simulink model "MotorSysFin"  (R2019a)
settings: Solver=VariableStepAuto  StartTime=0.0  StopTime=10  RelTol=1e-3
libraries: fuzblock x2, simulink x1
settings Model: Creator=936305695  LastModifiedBy=936305695
settings SolverCC: AlgebraicLoopSolver=LineSearch

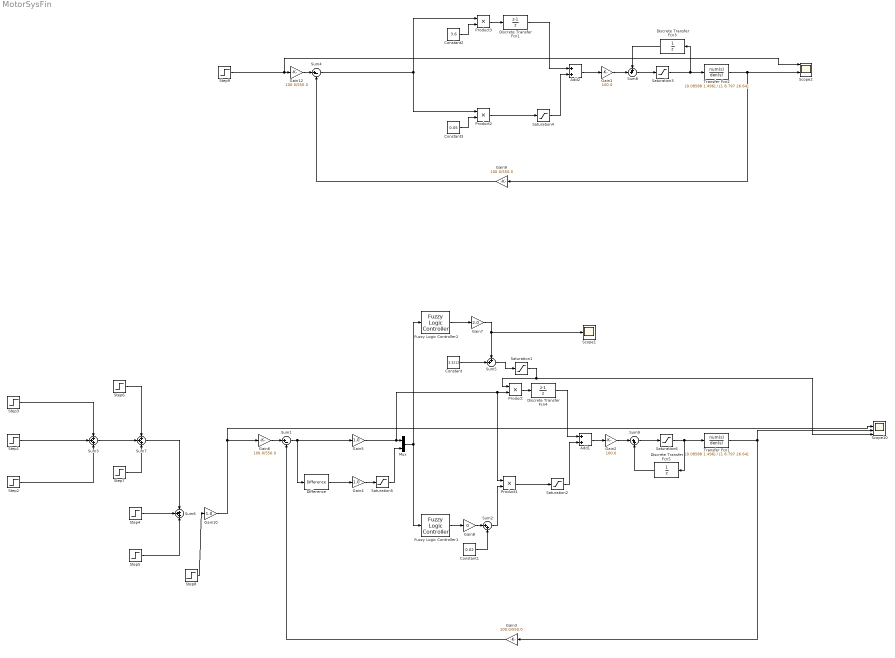
== system MotorSysFin ==
  Add1 : Sum
  Add2 : Sum
  Constant : Constant  Value=3.3212
  Constant1 : Constant  Value=0.02  SampleTime=0.002
  Constant2 : Constant  Value=3.6
  Constant3 : Constant  Value=0.05
  Difference : simulink/Discrete/Difference  ICPrevInput=0.0  OutMin=[]  OutMax=[]  OutDataType=fixdt(1, 16)  OutScaling=2^-10  DoSatur=off
  Discrete Transfer Fcn1 : DiscreteTransferFcn  Numerator=[1 -1]  Denominator=[1 0]  SampleTime=0.002
  Discrete Transfer Fcn3 : DiscreteTransferFcn  Denominator=[1 0]  SampleTime=0.002
  Discrete Transfer Fcn4 : DiscreteTransferFcn  Numerator=[1 -1]  Denominator=[1 0]  SampleTime=0.002
  Discrete Transfer Fcn5 : DiscreteTransferFcn  Denominator=[1 0]  SampleTime=0.002
  Fuzzy Logic Controller1 : fuzblock/Fuzzy Logic  Controller  FIS=mFuzzyKi  OutputSampleNumber=101  DataType=double  FuzzifiedInputs=off  RuleFiringStrengths=off  RuleOutputs=off  AggregatedOutputs=off  SimulateUsing=Interpreted execution  OutOfRangeInputValueMessage=warning  NoRuleFiredMessage=warning  EmptyOutputFuzzySetMessage=warning
  Fuzzy Logic Controller2 : fuzblock/Fuzzy Logic  Controller  FIS=mFuzzyKp  OutputSampleNumber=101  DataType=double  FuzzifiedInputs=off  RuleFiringStrengths=off  RuleOutputs=off  AggregatedOutputs=off  SimulateUsing=Interpreted execution  OutOfRangeInputValueMessage=warning  NoRuleFiredMessage=warning  EmptyOutputFuzzySetMessage=warning
  Gain1 : Gain  Gain=100.0
  Gain10 : Gain  Gain=1.0
  Gain{3,6,9,12} (4 alike) : Gain  Gain=100.0/550.0
  Gain2 : Gain  Gain=100.0
  Gain4 : Gain  Gain=1.0
  Gain5 : Gain  Gain=1.0
  Gain7 : Gain  Gain=2.0
  Gain8 : Gain  Gain=0
  Mux : Mux  Inputs=2
  Product{,1..3} (4 alike) : Product
  Saturation1 : Saturate  UpperLimit=20.0  LowerLimit=1.0
  Saturation2 : Saturate  UpperLimit=1.2  LowerLimit=-1.2
  Saturation3 : Saturate  UpperLimit=10000.0  LowerLimit=-10000.0
  Saturation4 : Saturate  UpperLimit=100  LowerLimit=-100
  Saturation5 : Saturate  UpperLimit=20.0  LowerLimit=-20.0
  Saturation6 : Saturate  UpperLimit=10000.0  LowerLimit=-10000.0
  Scope1 : Scope
  Scope10 : Scope  NumInputPorts=4
  Scope2 : Scope  NumInputPorts=4
  Step1 : Step  After=150  SampleTime=0
  Step2 : Step  Time=2  After=-100  SampleTime=0
  Step3 : Step  Time=3  After=100  SampleTime=0
  Step4 : Step  Time=6  After=-100  SampleTime=0
  Step5 : Step  Time=7  After=-50  SampleTime=0
  Step6 : Step  Time=4  After=-50  SampleTime=0
  Step7 : Step  Time=5  After=100  SampleTime=0
  Step8 : Step  After=150  SampleTime=0.002
  Step9 : Step  After=150  SampleTime=0.002
  Sum1 : Sum  Inputs=|+-
  Sum2 : Sum  Inputs=|++
  Sum3 : Sum  Inputs=+++
  Sum4 : Sum  Inputs=|+-
  Sum5 : Sum  Inputs=++|
  Sum6 : Sum  Inputs=+++
  Sum7 : Sum  Inputs=+++
  Sum8 : Sum  Inputs=++|
  Sum9 : Sum  Inputs=|++
  Transfer Fcn1 : TransferFcn  Numerator=[0.08588 1.496]  Denominator=[1 8.797 26.64]
  Transfer Fcn2 : TransferFcn  Numerator=[0.08588 1.496]  Denominator=[1 8.797 26.64]
  wires:
  Saturation2/1 -> Add1/2
  Product1/1 -> Saturation2/1
  Discrete Transfer Fcn4/1 -> Add1/1
  Transfer Fcn1/1 -> Scope10/3, Gain3/1
  Gain3/1 -> Sum1/2
  Sum1/1 -> Gain5/1, Difference/1
  Gain6/1 -> Sum1/1
  Mux/1 -> Fuzzy Logic Controller2/1, Fuzzy Logic Controller1/1
  Fuzzy Logic Controller2/1 -> Gain7/1
  Gain7/1 -> Sum5/1, Scope1/1
  Fuzzy Logic Controller1/1 -> Gain8/1
  Discrete Transfer Fcn1/1 -> Add2/1
  Product2/1 -> Saturation4/1
  Transfer Fcn2/1 -> Scope2/3, Gain9/1
  Gain9/1 -> Sum4/2
  Saturation4/1 -> Add2/2
  Gain12/1 -> Sum4/1
  Difference/1 -> Gain4/1
  Constant/1 -> Sum5/2
  Product/1 -> Discrete Transfer Fcn4/1
  Constant1/1 -> Sum2/2
  Gain8/1 -> Sum2/1
  Sum2/1 -> Product1/2
  Sum4/1 -> Product3/1, Product2/1
  Product3/1 -> Discrete Transfer Fcn1/1
  Gain4/1 -> Saturation5/1
  Gain10/1 -> Scope10/2, Gain6/1
  Saturation5/1 -> Mux/2
  Gain5/1 -> Product1/1, Product/2, Mux/1
  Step2/1 -> Sum3/3
  Step1/1 -> Sum3/2
  Step3/1 -> Sum3/1
  Step5/1 -> Sum6/3
  Step4/1 -> Sum6/2
  Sum3/1 -> Sum7/2
  Sum7/1 -> Sum6/1
  Step6/1 -> Sum7/1
  Step7/1 -> Sum7/3
  Sum5/1 -> Saturation1/1
  Saturation1/1 -> Scope10/4, Product/1
  Saturation3/1 -> Discrete Transfer Fcn3/1, Transfer Fcn2/1
  Add2/1 -> Gain1/1
  Gain1/1 -> Sum8/2
  Discrete Transfer Fcn3/1 -> Sum8/1
  Sum8/1 -> Saturation3/1
  Add1/1 -> Gain2/1
  Saturation6/1 -> Discrete Transfer Fcn5/1, Transfer Fcn1/1
  Sum9/1 -> Saturation6/1
  Gain2/1 -> Sum9/1
  Discrete Transfer Fcn5/1 -> Sum9/2
  Step8/1 -> Gain10/1
  Constant2/1 -> Product3/2
  Constant3/1 -> Product2/2
  Step9/1 -> Scope2/1, Gain12/1
